simulink model "MIMO_scan_r2016b"  (R2016b)
settings: Solver=FixedStepDiscrete  StartTime=0.0  StopTime=15  FixedStep=50e-6  RelTol=1e-3
libraries: powerlib x1
settings Model: Creator=anony  LastModifiedBy=anony

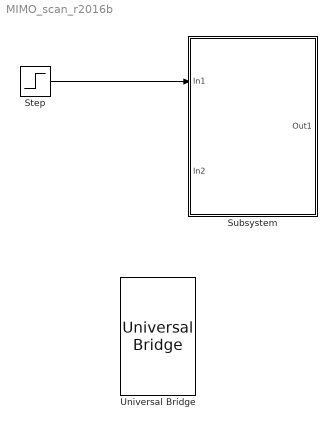
== system MIMO_scan_r2016b ==
  Step : Step  SampleTime=0
  Subsystem : Subsystem  mask{var_gui_external=External, var_freq_begin=0, var_freq_end=0, var_freq_step=0, var_freq_inject_amp=0, var_pos_or_neg_seq=Positive Sequence}
      mask prompts: var_gui_external "Set Parameters using GUI or External"; var_freq_begin "FreqBegin"; var_freq_end "FreqEnd"; var_freq_step "FreqStep"; var_freq_inject_amp "FreqInjectAmp"; var_pos_or_neg_seq "Positve or Negative Sequence"
      mask init:
      | block = find_system(gcb,...
      |           'LookUnderMasks','on',...
      |           'FollowLinks','on','Name','In2');
      | % p=Simulink.Mask.get(gcb);
      | switch var_gui_external
      |     case 1
      |       if ~isempty(block)
      |         delete_block(block);
      |       end
      | %       p.getDialogControl('para_group_gui_setting_zone').Visible='on';
      |     case 2
      |         if isempty(block)
      |             add_block('built-in/Inport',[gcb,'/In2']);
      |         end
      | %         p.getDialogControl('para_group_gui_setting_zone').Visible='off';
      | end % switch
      mask TypeOptions var_gui_external: GUI | External
      mask TypeOptions var_pos_or_neg_seq: Positive Sequence | Negative Sequence | Frequency Coupling Step1 | Frequency Coupling Step2
      mask DialogControl para_group_gui_setting_zone Prompt: GUI Setting Zone
  Universal Bridge : powerlib/Power Electronics/Universal Bridge  Arms=3  SnubberResistance=1e5  SnubberCapacitance=inf  Device=Thyristors  Ron=1e-3  Lon=0  ForwardVoltages="[  0  0  ]"  ForwardVoltage=0  GTOparameters=[ 10e-6 , 20e-6 ]  IGBTparameters=[ 1e-6 , 2e-6 ]  Measurements=None  Measurements_2=None  converterType=Rectifier
  wires:
  Step/1 -> Subsystem/1(In1)

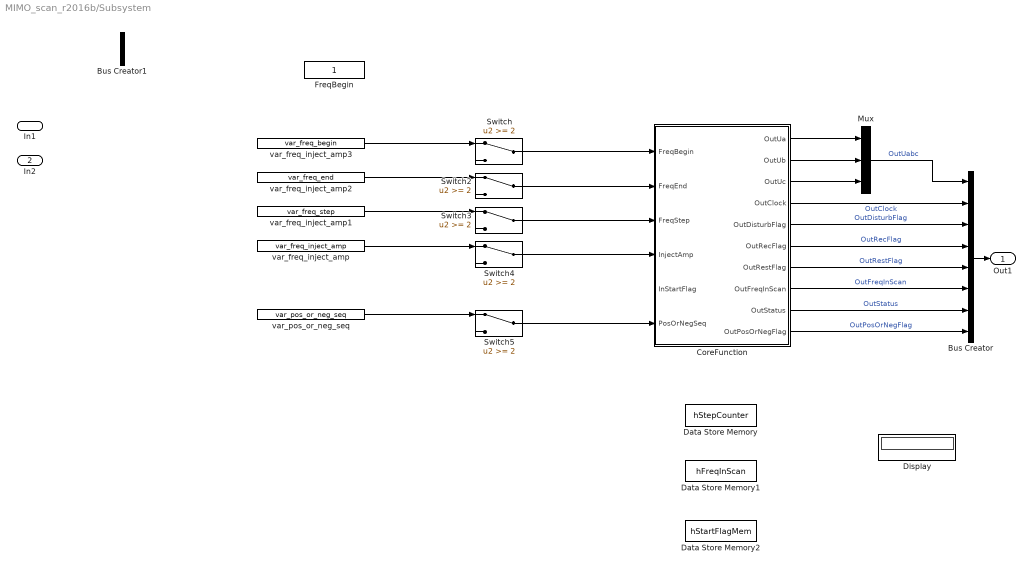
== system MIMO_scan_r2016b/Subsystem ==
  In1 : Inport
  In2 : Inport  Port=2
  Bus Creator : BusCreator  Inputs=8
  Bus Creator1 : BusCreator  Inputs=2
  CoreFunction : MATLAB Function  TreatAsAtomicUnit=on
  Data Store Memory : DataStoreMemory  DataStoreName=hStepCounter  ReadBeforeWriteMsg=warning  WriteAfterWriteMsg=warning  WriteAfterReadMsg=warning  ShowAdditionalParam=off  OutDataTypeStr=int32
  Data Store Memory1 : DataStoreMemory  DataStoreName=hFreqInScan  ReadBeforeWriteMsg=warning  WriteAfterWriteMsg=warning  WriteAfterReadMsg=warning  ShowAdditionalParam=off  OutDataTypeStr=double
  Data Store Memory2 : DataStoreMemory  DataStoreName=hStartFlagMem  ReadBeforeWriteMsg=warning  WriteAfterWriteMsg=warning  WriteAfterReadMsg=warning  ShowAdditionalParam=off  OutDataTypeStr=int32
  Display : Display
  FreqBegin : Constant
  Mux : Mux  Inputs=3
  Switch{,2..5} (5 alike) : Switch  Threshold=2
  var_freq_inject_amp : Constant  Value=var_freq_inject_amp
  var_freq_inject_amp1 : Constant  Value=var_freq_step
  var_freq_inject_amp2 : Constant  Value=var_freq_end
  var_freq_inject_amp3 : Constant  Value=var_freq_begin
  var_pos_or_neg_seq : Constant  Value=var_pos_or_neg_seq
  Out1 : Outport
  wires:
  CoreFunction/8(OutFreqInScan) -> Bus Creator/6  "OutFreqInScan"
  CoreFunction/7(OutRestFlag) -> Bus Creator/5  "OutRestFlag"
  CoreFunction/5(OutDisturbFlag) -> Bus Creator/3  "OutDisturbFlag"
  CoreFunction/6(OutRecFlag) -> Bus Creator/4  "OutRecFlag"
  CoreFunction/9(OutStatus) -> Bus Creator/7  "OutStatus"
  CoreFunction/4(OutClock) -> Bus Creator/2  "OutClock"
  Bus Creator/1 -> Out1/1
  CoreFunction/10(OutPosOrNegFlag) -> Bus Creator/8  "OutPosOrNegFlag"
  Mux/1 -> Bus Creator/1  "OutUabc"
  CoreFunction/1(OutUa) -> Mux/1
  CoreFunction/3(OutUc) -> Mux/3
  CoreFunction/2(OutUb) -> Mux/2
  Switch/1 -> CoreFunction/1(FreqBegin)
  Switch5/1 -> CoreFunction/6(PosOrNegSeq)
  var_pos_or_neg_seq/1 -> Switch5/1
  var_freq_inject_amp/1 -> Switch4/1
  var_freq_inject_amp2/1 -> Switch2/1
  var_freq_inject_amp1/1 -> Switch3/1
  Switch2/1 -> CoreFunction/2(FreqEnd)
  Switch3/1 -> CoreFunction/3(FreqStep)
  Switch4/1 -> CoreFunction/4(InjectAmp)
  var_freq_inject_amp3/1 -> Switch/1

== matlab function MIMO_scan_r2016b/Subsystem/CoreFunction ==
  data: FreqBegin input; OutUa output; FreqEnd input; FreqStep input; InjectAmp input; InStartFlag input; PosOrNegSeq input; OutUb output; OutUc output; OutClock output; OutDisturbFlag output; OutRecFlag output; OutRestFlag output; OutFreqInScan output; OutStatus output; OutPosOrNegFlag output; hStepCounter data_store_memory; hFreqInScan data_store_memory; hStartFlagMem data_store_memory
function [OutUa, OutUb, OutUc, ...
    OutClock, OutDisturbFlag, OutRecFlag, OutRestFlag, ...
    OutFreqInScan, OutStatus, OutPosOrNegFlag] = ...
    fcn(FreqBegin, FreqEnd, FreqStep, InjectAmp, InStartFlag, PosOrNegSeq)

global hStepCounter;
global hFreqInScan; 
global hStartFlagMem;
SAMPLE_FREQ = 1/50e-6;
SAMPLE_TIME = 1/SAMPLE_FREQ;

T_DISTURB	= 2 * SAMPLE_FREQ;
T_REC 		= 1 * SAMPLE_FREQ;
T_REST 		= 1 * SAMPLE_FREQ;

clock_t		= 0;
start_flag	= 0;
status_code	= 0;
ua			= 0; 
ub			= 0; 
uc			= 0;
omega		= 0;
disturb_flag = 0;
rec_flag    = 0;
rest_flag   = 0;

start_flag = InStartFlag;
	if (start_flag >= 1 && hFreqInScan >= FreqBegin)
		if (hStartFlagMem == 0)
			hFreqInScan = FreqBegin;
			status_code = -1;
        end
		
		if ((hFreqInScan >= FreqBegin) && (hFreqInScan <= FreqEnd))
			status_code = 1;
			if (hStepCounter <= (T_DISTURB - T_REC))
				disturb_flag = 1;
				rec_flag = 0;
				rest_flag = 0;
				hStepCounter = hStepCounter + 1;
            elseif ((hStepCounter > (T_DISTURB - T_REC)) && (hStepCounter <= T_DISTURB))
				disturb_flag = 1;
				rec_flag = 1;
				rest_flag = 0;
				hStepCounter = hStepCounter + 1;
            elseif ((hStepCounter > T_DISTURB) && hStepCounter <= (T_DISTURB + T_REST))
				disturb_flag = 0;
				rec_flag = 0;
				rest_flag = 1;
				hStepCounter = hStepCounter + 1;
            else
				hStepCounter = int32(0);
				hFreqInScan = hFreqInScan + FreqStep;
				ua = 0; ub = 0; uc = 0;
            end

			if (disturb_flag == 1) 
				clock_t = double(hStepCounter) * SAMPLE_TIME;
				omega = 2.0 * hFreqInScan * pi;
				if (PosOrNegSeq == 1)
					ua = InjectAmp * sin(omega * clock_t);
					ub = InjectAmp * sin(omega * clock_t - 2.0*pi/3.0);
					uc = InjectAmp * sin(omega * clock_t + 2.0*pi/3.0);
				
                elseif (PosOrNegSeq == 2)
					ua = InjectAmp * sin(omega * clock_t);
					ub = InjectAmp * sin(omega * clock_t + 2.0*pi/3.0);
					uc = InjectAmp * sin(omega * clock_t - 2.0*pi/3.0);
                elseif (PosOrNegSeq == 3)
                    1;
                elseif (PosOrNegSeq == 4)
                end
			else 
				ua = 0; ub = 0; uc = 0;
            end
			
		
        elseif (hFreqInScan > FreqEnd ) 
			status_code = 2;
			hFreqInScan = 0;
			ua = 0; ub = 0; uc = 0;
		
		else 
			status_code = 3;
        end

    else
		if (hStartFlagMem == 0)
			hFreqInScan = FreqBegin;
			status_code = -1;
        else
			status_code = 0;
			disturb_flag = 0;
			rec_flag = 0;
			rest_flag = 0;
			hStepCounter = int32(0);
			clock_t = double(hStepCounter) * SAMPLE_TIME;
			ua = 0; ub = 0; uc = 0;
        end
    end

		
		
	hStartFlagMem = int32(start_flag);  % record start_flag
	OutUa = ua;
	OutUb = ub;
	OutUc = uc;

	OutStatus = status_code;
	OutFreqInScan = hFreqInScan;
	OutClock = clock_t;
	OutDisturbFlag = disturb_flag;
	OutRecFlag = rec_flag;
	OutRestFlag = rest_flag;
    OutPosOrNegFlag = PosOrNegSeq;
end
